simulink model "ClosedLoopSysLQR"  (R2025b)
settings: Solver=FixedStepAuto  StartTime=0.00  StopTime=60  FixedStep=Ts  RelTol=1e-5  EnableMultiTasking=on
undefined symbols (not defined in the file or in its folder): amp_sat_u, DAC_lim_u, F_e_real, g_real, J_E_real, J_Psi_real, J_Theta_real, kd, ks, l1, l2, l3, m1, m2, sys_fan, Ts, U_e_real
settings Model: VariantConfigurationObject=var_config_vcdo  Creator=bjones  LastModifiedBy=leeta
settings SolverCC: AlgebraicLoopSolver=TrustRegion
settings DataIOCC: SaveFormat=Array  SignalLoggingSaveFormat=ModelDataLogs  ReturnWorkspaceOutputs=off
settings OptimizationCC: BlockReduction=off  BooleanDataType=off  ExpressionDepthLimit=2147483647.0  LifeSpan=inf
settings DebuggingCC: SaveWithParameterizedLinksMsg=none  MergeDetectMultiDrivingBlocksExec=none  SignalResolutionControl=TryResolveAllWithWarning  MultiTaskDSMMsg=warning  MultiTaskCondExecSysMsg=none  FcnCallInpInsideContextMsg=warning  UnconnectedInputMsg=warning  UnconnectedOutputMsg=warning  UnconnectedLineMsg=warning  StateNameClashWarn=warning  SFUnexpectedBacktrackingDiag=warning  SFNoUnconditionalDefaultTransitionDiag=warning  SFExecutionAtInitializationDiag=none  ArithmeticOperatorsInVariantConditions=warning
settings HardwareCC: ProdBitPerPointer=32.0  ProdBitPerSizeT=32.0  ProdBitPerPtrDiffT=32.0  ProdLargestAtomicFloat=None  ProdIntDivRoundTo=Undefined  ProdEndianess=Unspecified  ProdWordSize=32.0  ProdHWDeviceType=32-bit Generic  TargetUnknown=on
settings ModelReferenceCC: EnableRefExpFcnMdlSchedulingChecks=on  PropagateSignalLabelsOutOfModel=off
settings SFSimCC: SimUseLocalCustomCode=off  CustomCodeUndefinedFunction=UseInterfaceOnly
settings RTWCC: RTWUseLocalCustomCode=off  GPUComputeCapability=3.5
settings CodeAppCC: StateflowObjectComments=on
settings GRTTargetCC: TargetLangStandard=C89/C90 (ANSI)  CombineOutputUpdateFcns=off  GRTInterface=on
settings ConfigComp: CovMetricSettings=dw  CovSaveCumulativeToWorkspaceVar=on  CovSaveSingleToWorkspaceVar=on  CovExternalEMLEnable=off  CovSFcnEnable=off

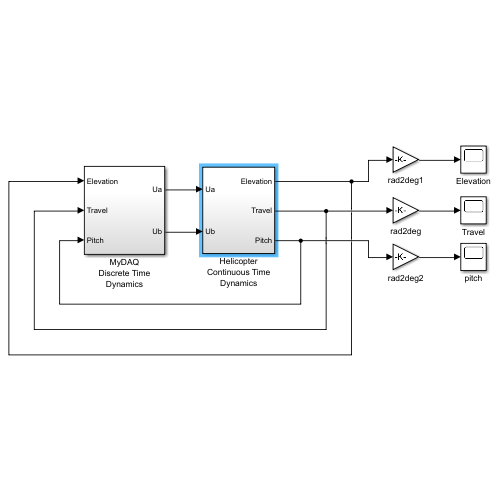
[thumbnail: Simulink's stored preview of the top-level diagram]
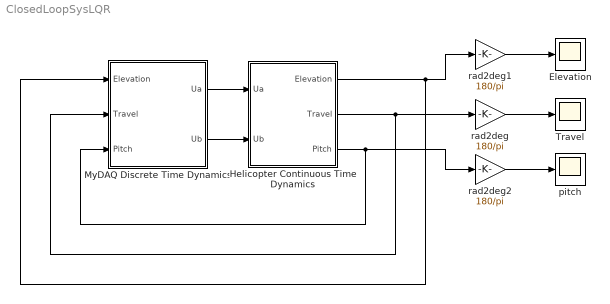
== system ClosedLoopSysLQR ==
  Elevation : Scope
      settings: TimeSpan=60  ActiveDisplayYMinimum=-112.71502718271525  ActiveDisplayYMaximum=79.814511512571656  DataLoggingVariableName=elev
  Helicopter Continuous Time Dynamics : Subsystem
  MyDAQ Discrete Time Dynamics : Subsystem
  Travel : Scope
      settings: TimeSpan=60  ActiveDisplayYMinimum=-5472.0887039350109  ActiveDisplayYMaximum=608.29454719906641  DataLoggingVariableName=trav
  pitch : Scope
      settings: TimeSpan=60  ActiveDisplayYMinimum=-104.48552614092141  ActiveDisplayYMaximum=197.22827580727838  DataLoggingVariableName=pitch
  rad2deg : Gain  Gain=180/pi  SaturateOnIntegerOverflow=on  OutDataTypeStr=Inherit: Same as input  ParamDataTypeStr=Inherit: Same as input
  rad2deg1 : Gain  Gain=180/pi  SaturateOnIntegerOverflow=on  OutDataTypeStr=Inherit: Same as input  ParamDataTypeStr=Inherit: Same as input
  rad2deg2 : Gain  Gain=180/pi  SaturateOnIntegerOverflow=on  OutDataTypeStr=Inherit: Same as input  ParamDataTypeStr=Inherit: Same as input
  wires:
  rad2deg/1 -> Travel/1
  rad2deg1/1 -> Elevation/1
  Helicopter Continuous Time Dynamics/2(Travel) -> MyDAQ Discrete Time Dynamics/2(Travel), rad2deg/1
  Helicopter Continuous Time Dynamics/1(Elevation) -> rad2deg1/1, MyDAQ Discrete Time Dynamics/1(Elevation)
  rad2deg2/1 -> pitch/1
  Helicopter Continuous Time Dynamics/3(Pitch) -> rad2deg2/1, MyDAQ Discrete Time Dynamics/3(Pitch)
  MyDAQ Discrete Time Dynamics/1(Ua) -> Helicopter Continuous Time Dynamics/1(Ua)
  MyDAQ Discrete Time Dynamics/2(Ub) -> Helicopter Continuous Time Dynamics/2(Ub)

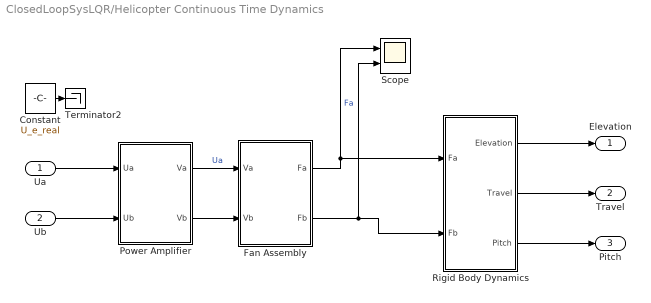
== system ClosedLoopSysLQR/Helicopter Continuous Time Dynamics ==
  Ua : Inport
  Ub : Inport  Port=2
  Constant : Constant  Value=U_e_real
  Fan Assembly : Subsystem
  Power Amplifier : Subsystem
  Rigid Body Dynamics : Subsystem
  Scope : Scope  NumInputPorts=2
      settings: ActiveDisplayYMinimum=-0.011433918489376946  ActiveDisplayYMaximum=0.029929551024525429  DataLoggingVariableName=ScopeData5
  Terminator2 : Terminator
  Elevation : Outport
  Travel : Outport  Port=2
  Pitch : Outport  Port=3
  wires:
  Power Amplifier/1(Va) -> Fan Assembly/1(Va)  "Ua"
  Power Amplifier/2(Vb) -> Fan Assembly/2(Vb)
  Rigid Body Dynamics/1(Elevation) -> Elevation/1
  Rigid Body Dynamics/3(Pitch) -> Pitch/1
  Rigid Body Dynamics/2(Travel) -> Travel/1
  Fan Assembly/1(Fa) -> Rigid Body Dynamics/1(Fa), Scope/1  "Fa"
  Fan Assembly/2(Fb) -> Scope/2, Rigid Body Dynamics/2(Fb)
  Ub/1 -> Power Amplifier/2(Ub)
  Constant/1 -> Terminator2/1
  Ua/1 -> Power Amplifier/1(Ua)

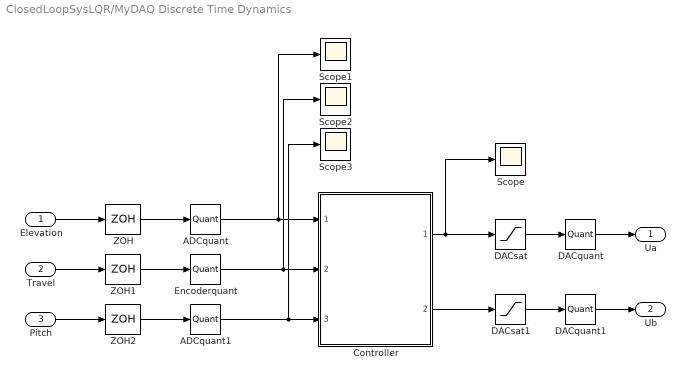
== system ClosedLoopSysLQR/MyDAQ Discrete Time Dynamics ==
  Elevation : Inport
  Travel : Inport  Port=2
  Pitch : Inport  Port=3
  ADCquant : Quantizer  QuantizationInterval=ADC_Vres  SampleTime=Ts
  ADCquant1 : Quantizer  QuantizationInterval=ADC_Vres  SampleTime=Ts
  Controller : Subsystem  ReferencedSubsystem=LQG_Integral
  DACquant : Quantizer  QuantizationInterval=DAC_Vres  SampleTime=Ts
  DACquant1 : Quantizer  QuantizationInterval=DAC_Vres  SampleTime=Ts
  DACsat : Saturate  UpperLimit=DAC_lim_u  LowerLimit=0  SampleTime=Ts
  DACsat1 : Saturate  UpperLimit=DAC_lim_u  LowerLimit=0  SampleTime=Ts
  Encoderquant : Quantizer  QuantizationInterval=Encoder_res  SampleTime=Ts
  Scope{,1..3} (4 alike) : Scope
      Scope settings: ActiveDisplayYMinimum=-2.6605476935057473  ActiveDisplayYMaximum=10.706688231224366
      Scope1 settings: ActiveDisplayYMinimum=-1.3085329717356646  ActiveDisplayYMaximum=1.8291802955314285  DataLoggingVariableName=ScopeData2
      Scope2 settings: ActiveDisplayYMinimum=-1  ActiveDisplayYMaximum=1
      Scope3 settings: ActiveDisplayYMinimum=-1  ActiveDisplayYMaximum=1  DataLoggingVariableName=ScopeData2
  ZOH : ZeroOrderHold  SampleTime=Ts
  ZOH1 : ZeroOrderHold  SampleTime=Ts
  ZOH2 : ZeroOrderHold  SampleTime=Ts
  Ua : Outport
  Ub : Outport  Port=2
  wires:
  Elevation/1 -> ZOH/1
  Travel/1 -> ZOH1/1
  DACquant/1 -> Ua/1
  DACquant1/1 -> Ub/1
  DACsat/1 -> DACquant/1
  DACsat1/1 -> DACquant1/1
  ZOH1/1 -> Encoderquant/1
  ZOH/1 -> ADCquant/1
  Pitch/1 -> ZOH2/1
  ZOH2/1 -> ADCquant1/1
  Controller/1 -> Scope/1, DACsat/1
  Controller/2 -> DACsat1/1
  ADCquant/1 -> Controller/1, Scope1/1
  Encoderquant/1 -> Controller/2, Scope2/1
  ADCquant1/1 -> Controller/3, Scope3/1

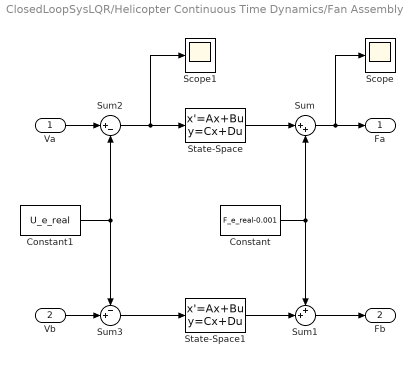
== system ClosedLoopSysLQR/Helicopter Continuous Time Dynamics/Fan Assembly ==
  Va : Inport
  Vb : Inport  Port=2
  Constant : Constant  Value=F_e_real-0.001
  Constant1 : Constant  Value=U_e_real
  Scope : Scope
      settings: ActiveDisplayYMinimum=-0.057263357526843334  ActiveDisplayYMaximum=0.03171902594878126
  Scope1 : Scope
      settings: ActiveDisplayYMinimum=-0.41466503024089013  ActiveDisplayYMaximum=0.34677059738963817  DataLoggingVariableName=ScopeData3
  State-Space : StateSpace  A=sys_fan.A  B=sys_fan.B  C=sys_fan.C  D=sys_fan.D  InitialCondition=0
  State-Space1 : StateSpace  A=sys_fan.A  B=sys_fan.B  C=sys_fan.C  D=sys_fan.D  InitialCondition=0
  Sum : Sum  Inputs=|++
  Sum1 : Sum  Inputs=++|
  Sum2 : Sum  Inputs=|+-
  Sum3 : Sum  Inputs=-+|
  Fa : Outport
  Fb : Outport  Port=2
  wires:
  Va/1 -> Sum2/1
  State-Space1/1 -> Sum1/2
  Sum/1 -> Scope/1, Fa/1
  Sum1/1 -> Fb/1
  Constant/1 -> Sum/2, Sum1/1
  Sum2/1 -> Scope1/1, State-Space/1
  Vb/1 -> Sum3/2
  Sum3/1 -> State-Space1/1
  Constant1/1 -> Sum3/1, Sum2/2
  State-Space/1 -> Sum/1

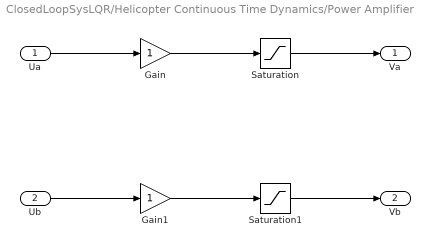
== system ClosedLoopSysLQR/Helicopter Continuous Time Dynamics/Power Amplifier ==
  Ua : Inport
  Ub : Inport  Port=2
  Gain : Gain
  Gain1 : Gain
  Saturation : Saturate  UpperLimit=amp_sat_u  LowerLimit=-amp_sat_u
  Saturation1 : Saturate  UpperLimit=amp_sat_u  LowerLimit=-amp_sat_u
  Va : Outport
  Vb : Outport  Port=2
  wires:
  Ua/1 -> Gain/1
  Gain/1 -> Saturation/1
  Saturation/1 -> Va/1
  Saturation1/1 -> Vb/1
  Gain1/1 -> Saturation1/1
  Ub/1 -> Gain1/1

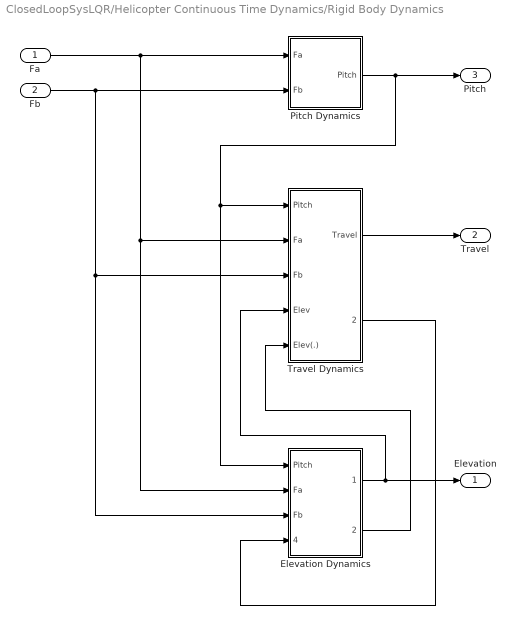
== system ClosedLoopSysLQR/Helicopter Continuous Time Dynamics/Rigid Body Dynamics ==
  Fa : Inport
  Fb : Inport  Port=2
  Elevation Dynamics : Subsystem
  Pitch Dynamics : Subsystem
  Travel Dynamics : Subsystem
  Elevation : Outport
  Travel : Outport  Port=2
  Pitch : Outport  Port=3
  wires:
  Fa/1 -> Pitch Dynamics/1(Fa), Travel Dynamics/2(Fa), Elevation Dynamics/2(Fa)
  Fb/1 -> Pitch Dynamics/2(Fb), Elevation Dynamics/3(Fb), Travel Dynamics/3(Fb)
  Travel Dynamics/1(Travel) -> Travel/1
  Elevation Dynamics/1(Elevation) -> Elevation/1, Travel Dynamics/4(Elev)
  Pitch Dynamics/1(Pitch) -> Travel Dynamics/1(Pitch), Elevation Dynamics/1(Pitch), Pitch/1
  Travel Dynamics/2(Travel(.)) -> Elevation Dynamics/4(Travel(.))
  Elevation Dynamics/2(Elevation(.)) -> Travel Dynamics/5(Elev(.))

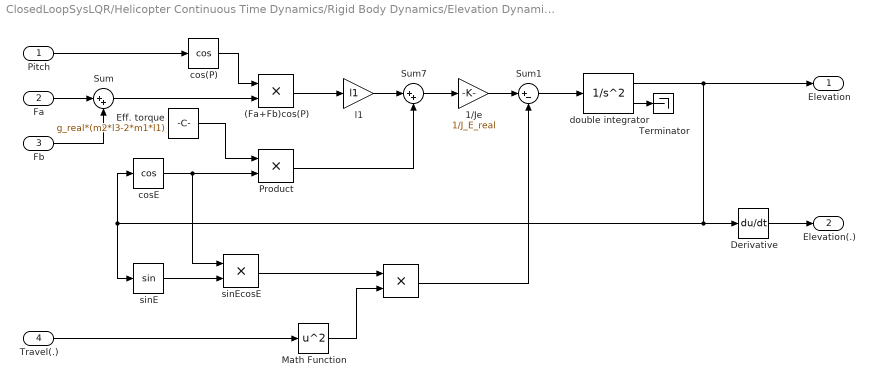
== system ClosedLoopSysLQR/Helicopter Continuous Time Dynamics/Rigid Body Dynamics/Elevation Dynamics ==
  Pitch : Inport
  Fa : Inport  Port=2
  Fb : Inport  Port=3
  Travel(.) : Inport  Port=4
  " " : Product  InputSameDT=on  RndMeth=Zero  SaturateOnIntegerOverflow=on  OutDataTypeStr=Inherit: Same as first input
  (Fa+Fb)cos(P) : Product  InputSameDT=on  RndMeth=Zero  SaturateOnIntegerOverflow=on  OutDataTypeStr=Inherit: Same as first input
  1/Je : Gain  Gain=1/J_E_real  SaturateOnIntegerOverflow=on  OutDataTypeStr=Inherit: Same as input  ParamDataTypeStr=Inherit: Same as input
  Derivative : Derivative
  Eff. torque : Constant  Value=g_real*(m2*l3-2*m1*l1)
  Math Function : Math  Operator=square  SignedPower=on
  Product : Product  InputSameDT=on  RndMeth=Zero  SaturateOnIntegerOverflow=on  OutDataTypeStr=Inherit: Same as first input
  Sum : Sum  Inputs=|++  InputSameDT=on  SaturateOnIntegerOverflow=on  OutDataTypeStr=Inherit: Same as first input
  Sum1 : Sum  Inputs=|+-  InputSameDT=on  SaturateOnIntegerOverflow=on  OutDataTypeStr=Inherit: Same as first input
  Sum7 : Sum  Inputs=|++  InputSameDT=on  SaturateOnIntegerOverflow=on  OutDataTypeStr=Inherit: Same as first input
  Terminator : Terminator
  cos(P) : Trigonometry  Operator=cos
  cosE : Trigonometry  Operator=cos
  double integrator : SecondOrderIntegrator  ICX=E0  LimitX=on  UpperLimitX=e_lim_u  LowerLimitX=e_lim_l  LimitDXDT=on  UpperLimitDXDT=2*pi  LowerLimitDXDT=-2*pi
  l1 : Gain  Gain=l1  SaturateOnIntegerOverflow=on  OutDataTypeStr=Inherit: Same as input  ParamDataTypeStr=Inherit: Same as input
  sinE : Trigonometry
  sinEcosE : Product  InputSameDT=on  RndMeth=Zero  SaturateOnIntegerOverflow=on  OutDataTypeStr=Inherit: Same as first input
  Elevation : Outport
  Elevation(.) : Outport  Port=2
  wires:
  double integrator/1 -> Elevation/1, sinE/1, cosE/1, Derivative/1
  Derivative/1 -> Elevation(.)/1
  double integrator/2 -> Terminator/1
  Pitch/1 -> cos(P)/1
  Fa/1 -> Sum/1
  Fb/1 -> Sum/2
  cos(P)/1 -> (Fa+Fb)cos(P)/1
  Sum/1 -> (Fa+Fb)cos(P)/2
  (Fa+Fb)cos(P)/1 -> l1/1
  l1/1 -> Sum7/1
  Sum7/1 -> 1/Je/1
  1/Je/1 -> Sum1/1
  Sum1/1 -> double integrator/1
  Travel(.)/1 -> Math Function/1
  Eff. torque/1 -> Product/1
  cosE/1 -> sinEcosE/1, Product/2
  sinE/1 -> sinEcosE/2
  sinEcosE/1 -> " "/1
  Math Function/1 -> " "/2
  Product/1 -> Sum7/2
  " "/1 -> Sum1/2

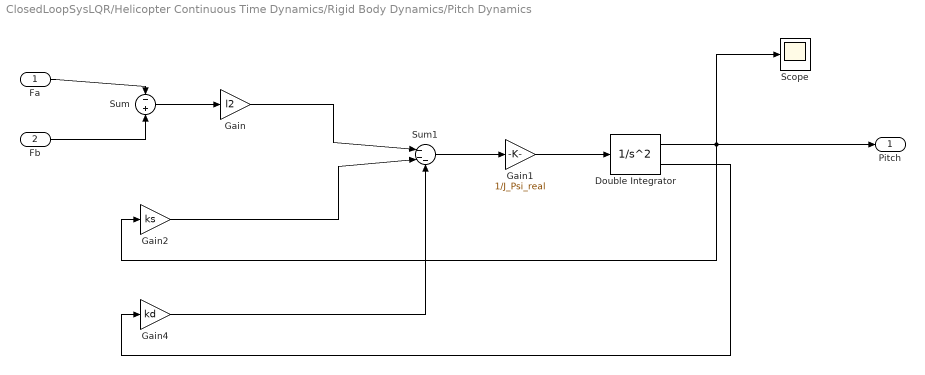
== system ClosedLoopSysLQR/Helicopter Continuous Time Dynamics/Rigid Body Dynamics/Pitch Dynamics ==
  Fa : Inport
  Fb : Inport  Port=2
  Double Integrator : SecondOrderIntegrator  ICX=P0  LimitX=on  UpperLimitX=p_lim_u  LowerLimitX=p_lim_l
  Gain : Gain  Gain=l2
  Gain1 : Gain  Gain=1/J_Psi_real
  Gain2 : Gain  Gain=ks
  Gain4 : Gain  Gain=kd
  Scope : Scope
      settings: ActiveDisplayYMinimum=-1  ActiveDisplayYMaximum=1  DataLoggingVariableName=ScopeData2
  Sum : Sum  Inputs=-+
  Sum1 : Sum  Inputs=|---
  Pitch : Outport
  wires:
  Fa/1 -> Sum/1
  Sum1/1 -> Gain1/1
  Fb/1 -> Sum/2
  Gain4/1 -> Sum1/3
  Double Integrator/2 -> Gain4/1
  Sum/1 -> Gain/1
  Gain2/1 -> Sum1/2
  Double Integrator/1 -> Pitch/1, Scope/1, Gain2/1
  Gain1/1 -> Double Integrator/1
  Gain/1 -> Sum1/1

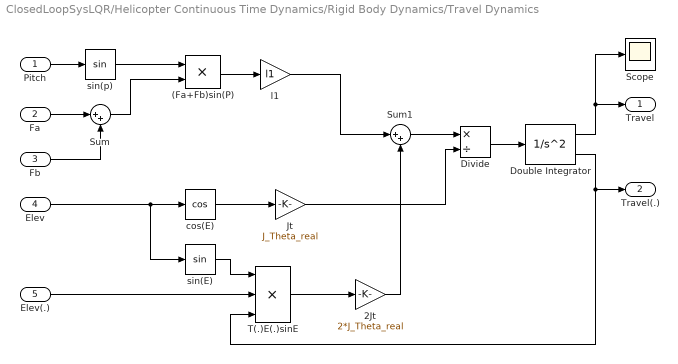
== system ClosedLoopSysLQR/Helicopter Continuous Time Dynamics/Rigid Body Dynamics/Travel Dynamics ==
  Pitch : Inport
  Fa : Inport  Port=2
  Fb : Inport  Port=3
  Elev : Inport  Port=4
  Elev(.) : Inport  Port=5
  (Fa+Fb)sin(P) : Product  InputSameDT=on  RndMeth=Zero  SaturateOnIntegerOverflow=on  OutDataTypeStr=Inherit: Same as first input
  2Jt : Gain  Gain=2*J_Theta_real  SaturateOnIntegerOverflow=on  OutDataTypeStr=Inherit: Same as input  ParamDataTypeStr=Inherit: Same as input
  Divide : Product  Inputs=*/
  Double Integrator : SecondOrderIntegrator  ICX=T0  UpperLimitX=1  LowerLimitX=0  LimitDXDT=on  UpperLimitDXDT=2  LowerLimitDXDT=-2
  Jt : Gain  Gain=J_Theta_real  SaturateOnIntegerOverflow=on  OutDataTypeStr=Inherit: Same as input  ParamDataTypeStr=Inherit: Same as input
  Scope : Scope
      settings: ActiveDisplayYMinimum=-95.505964844855143  ActiveDisplayYMaximum=10.61674267055176  DataLoggingVariableName=ScopeData4
  Sum : Sum  Inputs=|++  InputSameDT=on  SaturateOnIntegerOverflow=on  OutDataTypeStr=Inherit: Same as first input
  Sum1 : Sum  Inputs=|++  InputSameDT=on  SaturateOnIntegerOverflow=on  OutDataTypeStr=Inherit: Same as first input
  T(.)E(.)sinE : Product  Inputs=3  InputSameDT=on  RndMeth=Zero  SaturateOnIntegerOverflow=on  OutDataTypeStr=Inherit: Same as first input
  cos(E) : Trigonometry  Operator=cos
  l1 : Gain  Gain=l1  SaturateOnIntegerOverflow=on  OutDataTypeStr=Inherit: Same as input  ParamDataTypeStr=Inherit: Same as input
  sin(E) : Trigonometry
  sin(p) : Trigonometry
  Travel : Outport
  Travel(.) : Outport  Port=2
  wires:
  Double Integrator/1 -> Scope/1, Travel/1
  sin(p)/1 -> (Fa+Fb)sin(P)/1
  (Fa+Fb)sin(P)/1 -> l1/1
  Pitch/1 -> sin(p)/1
  Fa/1 -> Sum/1
  Fb/1 -> Sum/2
  Sum/1 -> (Fa+Fb)sin(P)/2
  Elev/1 -> cos(E)/1, sin(E)/1
  Double Integrator/2 -> Travel(.)/1, T(.)E(.)sinE/3
  sin(E)/1 -> T(.)E(.)sinE/1
  Elev(.)/1 -> T(.)E(.)sinE/2
  T(.)E(.)sinE/1 -> 2Jt/1
  2Jt/1 -> Sum1/2
  cos(E)/1 -> Jt/1
  Jt/1 -> Divide/2
  Sum1/1 -> Divide/1
  l1/1 -> Sum1/1
  Divide/1 -> Double Integrator/1
